simulink model "CCFE"  (R2025b)
settings: Solver=VariableStepAuto  StartTime=0.0  StopTime=20  RelTol=1e-3
settings Model: Creator=Asus  LastModifiedBy=Asus

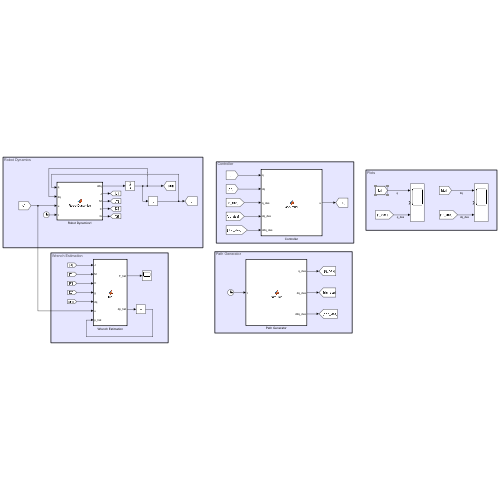
[thumbnail: Simulink's stored preview of the top-level diagram]
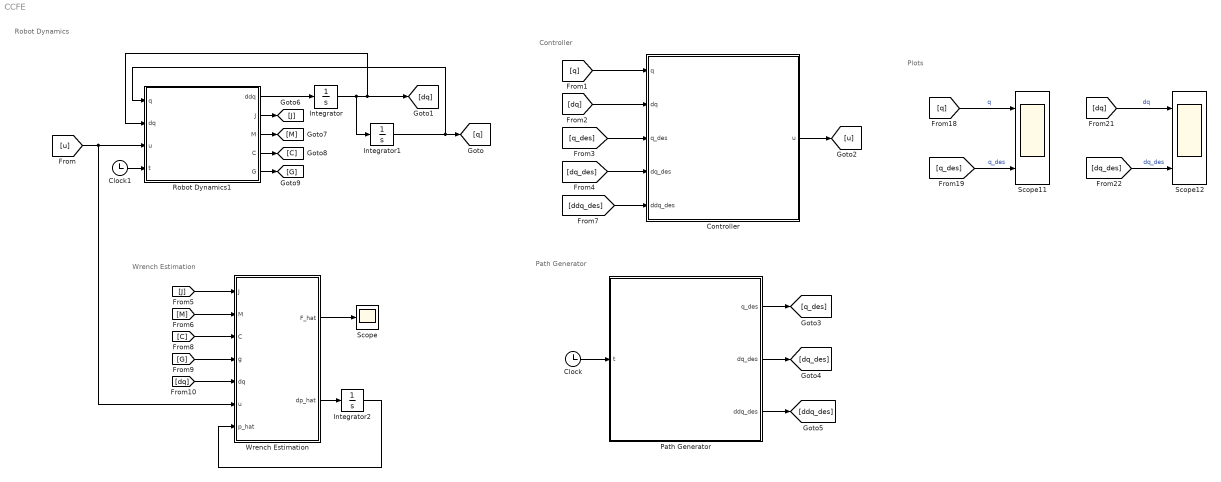
== system CCFE ==
  note: Plots
  note: Wrench Estimation
  note: Robot Dynamics
  note: Controller
  note: Path Generator
  Clock : Clock
  Clock1 : Clock
  Controller : MATLAB Function  TreatAsAtomicUnit=on
  Integrator : Integrator  InitialCondition=zeros(2, 1)
  Integrator1 : Integrator  InitialCondition=zeros(2, 1)
  Integrator2 : Integrator  InitialCondition=zeros(2, 1)
  Path Generator : MATLAB Function  TreatAsAtomicUnit=on
  Robot Dynamics1 : MATLAB Function  TreatAsAtomicUnit=on
  Scope : Scope
      settings: ActiveDisplayYMinimum=-6.2188637721728481  ActiveDisplayYMaximum=6.2189479950436457
  Scope11 : Scope  NumInputPorts=3
      settings: ActiveDisplayYMinimum=-0.66944442047593433  ActiveDisplayYMaximum=0.65256291478497264  DataLoggingVariableName=ScopeData5
  Scope12 : Scope  NumInputPorts=3
      settings: ActiveDisplayYMinimum=-2.2611222676056713  ActiveDisplayYMaximum=10.195386816907638  DataLoggingVariableName=ScopeData6
  Wrench Estimation : MATLAB Function  TreatAsAtomicUnit=on
  wires:
  [u] -> Wrench Estimation/6(u), Robot Dynamics1/3(u)
  [ddq_des] -> Controller/5(ddq_des)
  [q_des] -> Controller/3(q_des)
  [dq] -> Controller/2(dq)
  [q] -> Controller/1(q)
  [dq_des] -> Controller/4(dq_des)
  Path Generator/1(q_des) -> [q_des]
  Path Generator/3(ddq_des) -> [ddq_des]
  Path Generator/2(dq_des) -> [dq_des]
  Clock/1 -> Path Generator/1(t)
  Controller/1(u) -> [u]
  Clock1/1 -> Robot Dynamics1/4(t)
  [q] -> Scope11/1  "q"
  [q_des] -> Scope11/3  "q_des"
  [dq_des] -> Scope12/3  "dq_des"
  [dq] -> Scope12/1  "dq"
  Wrench Estimation/2(dp_hat) -> Integrator2/1
  Integrator2/1 -> Wrench Estimation/7(p_hat)
  Wrench Estimation/1(F_hat) -> Scope/1
  Robot Dynamics1/1(ddq) -> Integrator/1
  Integrator/1 -> Integrator1/1, Robot Dynamics1/2(dq), [dq]
  Integrator1/1 -> Robot Dynamics1/1(q), [q]
  Robot Dynamics1/2(J) -> [J]
  Robot Dynamics1/5(G) -> [G]
  Robot Dynamics1/4(C) -> [C]
  Robot Dynamics1/3(M) -> [M]
  [J] -> Wrench Estimation/1(J)
  [G] -> Wrench Estimation/4(g)
  [dq] -> Wrench Estimation/5(dq)
  [C] -> Wrench Estimation/3(C)
  [M] -> Wrench Estimation/2(M)

== matlab function CCFE/Controller ==
  data: q input; u output; dq input; q_des input; dq_des input; ddq_des input
function u = Controller(q, dq, q_des, dq_des, ddq_des)

    % Robot Params :
    m1 = 1;                 % mass of link 1
    m2 = 1;                 % mass of link 2
    l1 = 0.5;               % length of link 1
    lc1 = l1/2;             % length of center of mass link 1 
    l2 = 0.5;               % length of link 2
    lc2 = l2/2;             % length of center of mass link 2
    I1 = 1/12 * m1 * l1^2;  % inertia moment link 1
    I2 = 1/12 * m2 * l2^2;  % inertia moment link 2
    gravity = 9.81;         % gravity constant

    % M(q) Matrix :
    M11 = m1 * lc1^2 + I1 + m2 * (l1^2 + ...
        lc2^2 + 2 * l1 * lc2 * cos(q(2))) + I2;
    M12 = m2 * l1 * lc2 *cos(q(2)) + m2 * lc2^2 + I2;
    M21 = M12;
    M22 = m2 * lc2^2 + I2;
    M = [M11 M12; M21 M22];
     
    % G(q) Vector :
    G1 = m1 * lc1 * gravity * cos(q(1)) + m2 * gravity * ...
        (lc2 * cos(q(1) + q(2)) + l1 * cos(q(1)));
    G2 = m2 * lc2 * gravity * cos(q(1) + q(2));
    G = [G1; G2];
    
    % C(q,qdot) Matrix :
    h = m2 * l1 * lc2 * sin(q(2));
    C = [-h * dq(2), -h * (dq(1) + dq(2)); h * dq(1), 0];

    % error :
    q_tilde = q - q_des; dq_tilde = dq - dq_des;

    % controller gains :
    K1 = diag([100, 100]); K2 = diag([2500, 2500]);

    % inner loop :
    a_q = ddq_des - K1 * dq_tilde - K2 * q_tilde;

    % control law :
    u = M * a_q + C * dq + G;
    % u = zeros(2, 1);

end

== matlab function CCFE/Path Generator ==
  data: t input; q_des output; dq_des output; ddq_des output
function [q_des, dq_des, ddq_des] = PathGen(t)
    
    w = 0.2;
    A = 0.5;

    q_des   = A *       [ sin(w*t);  cos(w*t)];
    dq_des  = A * w *   [ cos(w*t); -sin(w*t)];
    ddq_des = A * w^2 * [-sin(w*t); -cos(w*t)];
    % q_des   = 0.5 * [1; 1];
    % dq_des  =       [0; 0];
    % ddq_des =       [0; 0];
    
end

== matlab function CCFE/Robot Dynamics1 ==
  data: q input; dq input; u input; ddq output; J output; t input; M output; C output; G output
function [ddq, J, M, C, G] = RobotDynamics(q, dq, u, t)
    
    % Robot Params :
    m1 = 1;                 % mass of link 1
    m2 = 1;                 % mass of link 2
    l1 = 0.5;               % length of link 1
    lc1 = l1/2;             % length of center of mass link 1 
    l2 = 0.5;               % length of link 2
    lc2 = l2/2;             % length of center of mass link 2
    I1 = 1/12 * m1 * l1^2;  % inertia moment link 1
    I2 = 1/12 * m2 * l2^2;  % inertia moment link 2
    gravity = 9.81;         % gravity constant

    % M(q) Matrix :
    M11 = m1 * lc1^2 + I1 + m2 * (l1^2 + ...
        lc2^2 + 2 * l1 * lc2 * cos(q(2))) + I2;
    M12 = m2 * l1 * lc2 *cos(q(2)) + m2 * lc2^2 + I2;
    M21 = M12;
    M22 = m2 * lc2^2 + I2;
    M = [M11 M12; M21 M22];
     
    % G(q) Vector :
    G1 = m1 * lc1 * gravity * cos(q(1)) + m2 * gravity * ...
        (lc2 * cos(q(1) + q(2)) + l1 * cos(q(1)));
    G2 = m2 * lc2 * gravity * cos(q(1) + q(2));
    G = [G1; G2];
    
    % C(q,qdot) Matrix :
    h = m2 * l1 * lc2 * sin(q(2));
    C = [-h * dq(2), -h * (dq(1) + dq(2)); h * dq(1), 0];

    % Jacobian Matrix :
    J = [-l1*sin(q(1)) - l2*sin(q(1)+q(2)), - l2*sin(q(1)+q(2));
          l1*cos(q(1)) + l2*cos(q(1)+q(2)),   l2*cos(q(1)+q(2));
          0                               ,   0                ;
          0                               ,   0                ;
          0                               ,   0                ;
          1                               ,   1                ];

    % wrench = zeros(6, 1);
    if t>2 && t<15
        wrench = [zeros(3, 1); 5*ones(3, 1)] * sin(t);
    else
        wrench = zeros(6, 1);
    end
    
    % robot dynamucis :
    ddq = M \ (u - C * dq - G - J' * wrench);

end

== matlab function CCFE/Wrench Estimation ==
  data: J input; M input; F_hat output; C input; g input; dq input; u input; p_hat input; dp_hat output
function [F_hat, dp_hat] = fcn(J, M, C, g, dq, u, p_hat)

    L = 10 * eye(2);

    tau_fric = zeros(2, 1);
    tau_bar = u + C' * dq - g - tau_fric;
    
    p = M * dq;
    dp_hat = tau_bar + L * (p - p_hat);
    
    tau_hat = - L * (p - p_hat);
    F_hat   = J' \ tau_hat;

end
